simulink model "Parameter_Estimation_of_DC_Motor"  (R2021b)
settings: Solver=VariableStepAuto  StartTime=0.0  StopTime=10.0  RelTol=1e-3
undefined symbols (not defined in the file): B_m, J_m, k_E, k_T, L_a, R_a
settings Model: Creator=AAwdallah  LastModifiedBy=AAwdallah

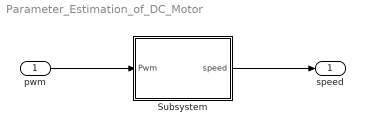
== system Parameter_Estimation_of_DC_Motor ==
  pwm : Inport
  Subsystem : Subsystem
  speed : Outport
  wires:
  pwm/1 -> Subsystem/1(Pwm)
  Subsystem/1(speed) -> speed/1

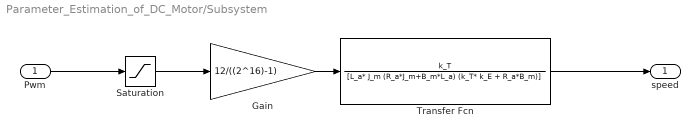
== system Parameter_Estimation_of_DC_Motor/Subsystem ==
  Pwm : Inport
  Gain : Gain  Gain=12/((2^16)-1)
  Saturation : Saturate  UpperLimit=(2^16)-1  LowerLimit=0
  Transfer Fcn : TransferFcn  Numerator=k_T  Denominator=[L_a* J_m (R_a*J_m+B_m*L_a) (k_T* k_E + R_a*B_m)]
  speed : Outport
  wires:
  Gain/1 -> Transfer Fcn/1
  Pwm/1 -> Saturation/1
  Saturation/1 -> Gain/1
  Transfer Fcn/1 -> speed/1
